simulink library "line_tracking_algorithm_atomic_sub_chart_library"  (R2013b)
settings: Solver=ode45  StartTime=0.0  StopTime=10.0  RelTol=1e-3
undefined symbols (not defined in the file): DiscIntNeverNeededParam, gcbh, realtime
libraries: legonxtlib x15, simulink x15
(part 1 of 2)
settings Model: Creator=mbiesiad  LastModifiedBy=menkh

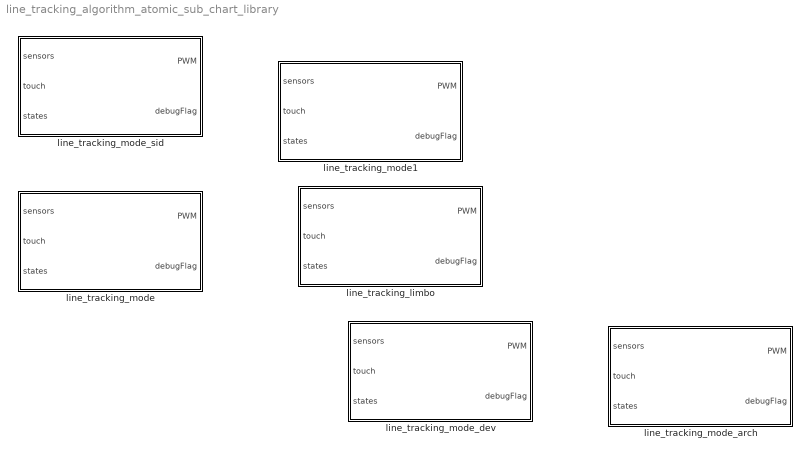
== system line_tracking_algorithm_atomic_sub_chart_library ==
  line_tracking_limbo : Stateflow chart  TreatAsAtomicUnit=on
  line_tracking_mode : Stateflow chart  TreatAsAtomicUnit=on
  line_tracking_mode1 : Stateflow chart  TreatAsAtomicUnit=on
  line_tracking_mode_arch : Stateflow chart  TreatAsAtomicUnit=on
  line_tracking_mode_dev : Stateflow chart  TreatAsAtomicUnit=on
  line_tracking_mode_sid : Stateflow chart  TreatAsAtomicUnit=on

== system line_tracking_algorithm_atomic_sub_chart_library/line_tracking_limbo/line_tracking_mode.DispTheta ==
  theta : Inport  OutDataTypeStr=double  PortDimensions=1
  f : TriggerPort  TriggerType=function-call
      settings: CopyFcn=Stateflow.SLINSF.SimulinkMan.removeBlockPreDeleteFcn  PreDeleteFcn=Stateflow.SLINSF.SimulinkMan.unsafePredeleteFcn
  Gain : Gain  Gain=10
  LCD : legonxtlib/LCD  slcdStr=Theta  slcdLine=2  slcdFormat=Decimal
  wires:
  theta/1 -> Gain/1
  Gain/1 -> LCD/1

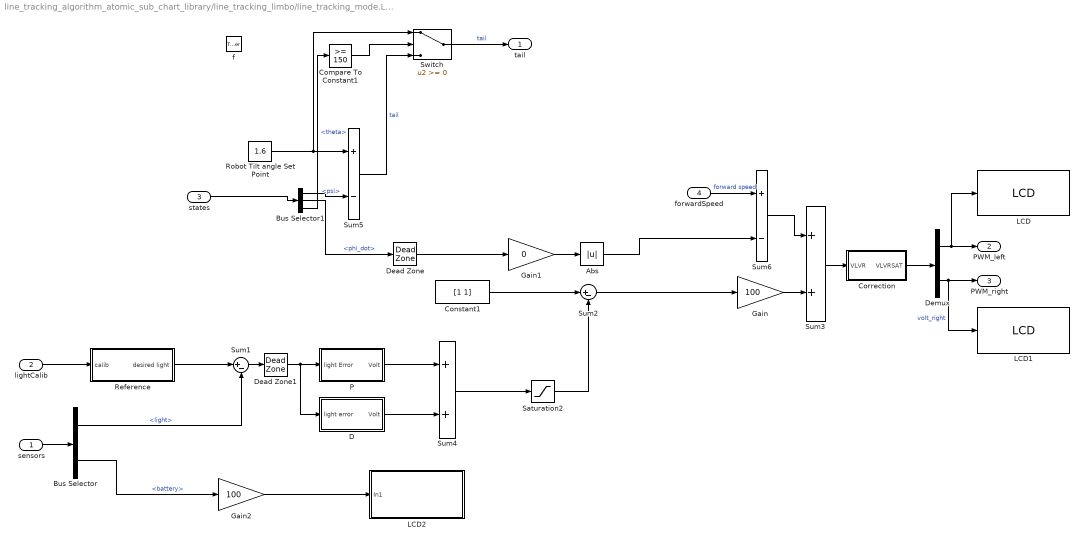
== system line_tracking_algorithm_atomic_sub_chart_library/line_tracking_limbo/line_tracking_mode.LineTrackAltFcn ==
  sensors : Inport  OutDataTypeStr=Bus: Sensors_Bus  PortDimensions=1
  lightCalib : Inport  Port=2  OutDataTypeStr=Bus: Light_Bus  PortDimensions=1
  states : Inport  Port=3  OutDataTypeStr=Bus: States_Bus  PortDimensions=1
  forwardSpeed : Inport  Port=4  OutDataTypeStr=single  PortDimensions=1
  f : TriggerPort  TriggerType=function-call
      settings: CopyFcn=Stateflow.SLINSF.SimulinkMan.removeBlockPreDeleteFcn  PreDeleteFcn=Stateflow.SLINSF.SimulinkMan.unsafePredeleteFcn
  Abs : Abs
  Bus Selector : BusSelector  OutputSignals=light,battery
  Bus Selector1 : BusSelector  OutputSignals=balancerStates.psi,phi_dot,balancerStates.theta
  Compare To Constant1 : simulink/Logic and Bit Operations/Compare To Constant  relop=>=  const=150  OutDataTypeStr=boolean
  Constant1 : Constant  Value=[1 1]  OutDataTypeStr=single
  Correction : Subsystem
  D : Subsystem
  Dead Zone : DeadZone  LowerValue=-3  UpperValue=3  SaturateOnIntegerOverflow=on
  Dead Zone1 : DeadZone  LowerValue=-0.1  UpperValue=0  SaturateOnIntegerOverflow=on
  Demux : Demux  Outputs=2
  Gain : Gain  Gain=100
  Gain1 : Gain  Gain=0
  Gain2 : Gain  Gain=100
  LCD : legonxtlib/LCD  slcdStr=VL  slcdLine=3  slcdFormat=Decimal
  LCD1 : legonxtlib/LCD  slcdStr=VR  slcdLine=4  slcdFormat=Decimal
  LCD2 : Subsystem  InitFcn=realtime.validateBlock('LEGO MINDSTORMS NXT', gcbh, '')  mask(LEGO MINDSTORMS NXT LCD){slcdStr=Battery, slcdLine=8, slcdFormat=Decimal}
      mask prompts: slcdStr "Display label (maximum  8 characters):"; slcdLine "Display at line:"; slcdFormat "Display format:"
      mask help: Displays the numeric value from the block input port. The display truncates the input value to show only the integer portion. Use Display at line parameter to select the row. Use Display format parameter to select the format of the number: decimal or hexadecimal.
      mask init:
      | realtime.internal.nxtLcdSysCallback;
      mask Help: eval('realtime.helpView(''LEGO MINDSTORMS NXT'', ''legonxtlibnxtlcd'')')
      mask TypeOptions slcdLine: 1 | 2 | 3 | 4 | 5 | 6 | 7 | 8
      mask TypeOptions slcdFormat: Decimal | Hex
      mask Display:
      | [data, map]=imread('LCD.gif');pic=ind2rgb(data,map);image(pic,[0.32 0.25 0.35 0.55]);
      | lineText = sprintf('Line %d', slcdLine);
      | text(0.5, 0.15, lineText, 'horizontalAlignment', 'center');
      | port_label('input', 1, '');
      | color('blue');
      | text(0.65, 0.87, 'LEGO', 'horizontalAlignment', 'left');
  P : Subsystem
  Reference : Subsystem
  Robot Tilt angle Set Point : Constant  Value=1.6  OutDataTypeStr=single
  Saturation2 : Saturate  UpperLimit=1  LowerLimit=0.45
  Sum1 : Sum  Inputs=|+-
  Sum2 : Sum  Inputs=|+-
  Sum3 : Sum
  Sum4 : Sum
  Sum5 : Sum  Inputs=+-
  Sum6 : Sum  Inputs=+-
  Switch : Switch
  tail : Outport  OutDataTypeStr=single  InitialOutput=0
  PWM_left : Outport  Port=2  OutDataTypeStr=single  InitialOutput=0
  PWM_right : Outport  Port=3  OutDataTypeStr=single  InitialOutput=0
  wires:
  Gain2/1 -> LCD2/1(In1)
  Bus Selector1/3 -> Compare To Constant1/1  "<theta>"
  Compare To Constant1/1 -> Switch/2
  Correction/1(VLVRSAT) -> Demux/1
  Sum3/1 -> Correction/1(VLVR)
  Abs/1 -> Sum6/2
  Bus Selector1/2 -> Dead Zone/1  "<phi_dot>"
  Gain1/1 -> Abs/1
  Sum6/1 -> Sum3/1
  Gain/1 -> Sum3/2
  Sum2/1 -> Gain/1
  forwardSpeed/1 -> Sum6/1  "forward speed"
  D/1(Volt) -> Sum4/2
  P/1(Volt) -> Sum4/1
  Reference/1(desired light) -> Sum1/1
  lightCalib/1 -> Reference/1(calib)
  Constant1/1 -> Sum2/1
  Robot Tilt angle Set Point/1 -> Switch/1, Sum5/1
  Bus Selector1/1 -> Sum5/2  "<psi>"
  states/1 -> Bus Selector1/1
  Sum4/1 -> Saturation2/1
  Sum1/1 -> Dead Zone1/1
  Saturation2/1 -> Sum2/2
  Bus Selector/1 -> Sum1/2  "<light>"
  sensors/1 -> Bus Selector/1
  Switch/1 -> tail/1  "tail"
  Demux/1 -> LCD/1, PWM_left/1
  Demux/2 -> LCD1/1, PWM_right/1  "volt_right"
  Dead Zone/1 -> Gain1/1
  Dead Zone1/1 -> P/1(light Error), D/1(light error)
  Sum5/1 -> Switch/3  "tail"
  Bus Selector/2 -> Gain2/1  "<battery>"

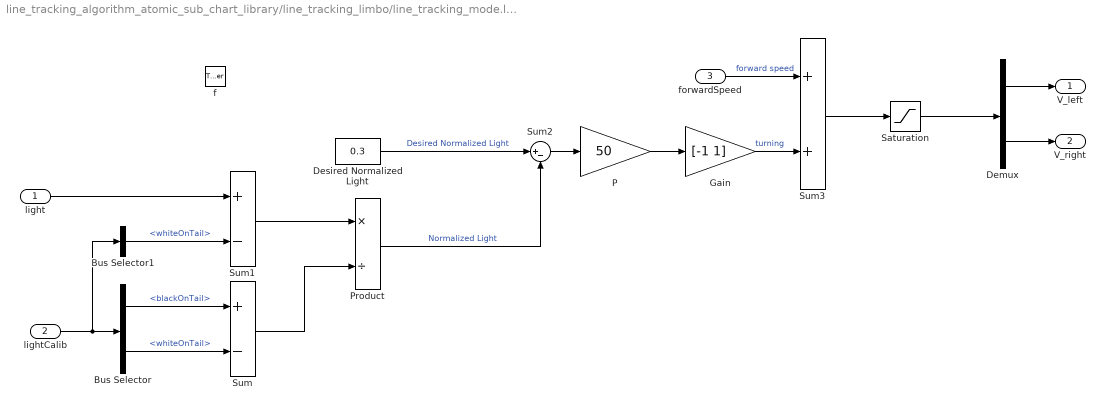
== system line_tracking_algorithm_atomic_sub_chart_library/line_tracking_limbo/line_tracking_mode.lineTrack ==
  light : Inport  OutDataTypeStr=single  PortDimensions=1
  lightCalib : Inport  Port=2  OutDataTypeStr=Bus: Light_Bus  PortDimensions=1
  forwardSpeed : Inport  Port=3  OutDataTypeStr=single  PortDimensions=1
  f : TriggerPort  TriggerType=function-call
      settings: CopyFcn=Stateflow.SLINSF.SimulinkMan.removeBlockPreDeleteFcn  PreDeleteFcn=Stateflow.SLINSF.SimulinkMan.unsafePredeleteFcn
  Bus Selector : BusSelector  OutputSignals=blackOnTail,whiteOnTail
  Bus Selector1 : BusSelector  OutputSignals=whiteOnTail
  Demux : Demux  Outputs=2
  Desired Normalized Light : Constant  Value=0.3  OutDataTypeStr=single
  Gain : Gain  Gain=[-1 1]
  P : Gain  Gain=50
  Product : Product  Inputs=*/
  Saturation : Saturate  UpperLimit=100  LowerLimit=-100  OutDataTypeStr=single
  Sum : Sum  Inputs=+-
  Sum1 : Sum  Inputs=+-
  Sum2 : Sum  Inputs=|+-
  Sum3 : Sum
  V_left : Outport  OutDataTypeStr=single  PortDimensions=1
  V_right : Outport  Port=2  OutDataTypeStr=single  PortDimensions=1
  wires:
  Saturation/1 -> Demux/1
  P/1 -> Gain/1
  Sum3/1 -> Saturation/1
  forwardSpeed/1 -> Sum3/1  "forward speed"
  Demux/2 -> V_right/1
  Demux/1 -> V_left/1
  Gain/1 -> Sum3/2  "turning"
  Sum2/1 -> P/1
  Desired Normalized Light/1 -> Sum2/1  "Desired Normalized Light"
  Product/1 -> Sum2/2  "Normalized Light"
  Sum1/1 -> Product/1
  Bus Selector1/1 -> Sum1/2  "<whiteOnTail>"
  light/1 -> Sum1/1
  Sum/1 -> Product/2
  Bus Selector/1 -> Sum/1  "<blackOnTail>"
  Bus Selector/2 -> Sum/2  "<whiteOnTail>"
  lightCalib/1 -> Bus Selector/1, Bus Selector1/1

== system line_tracking_algorithm_atomic_sub_chart_library/line_tracking_limbo/line_tracking_mode.tail_controller ==
  note: Could be improved, PI for example
  current : Inport  OutDataTypeStr=single  PortDimensions=1
  desired : Inport  Port=2  OutDataTypeStr=single  PortDimensions=1
  f : TriggerPort  TriggerType=function-call
      settings: CopyFcn=Stateflow.SLINSF.SimulinkMan.removeBlockPreDeleteFcn  PreDeleteFcn=Stateflow.SLINSF.SimulinkMan.unsafePredeleteFcn
  Gain : Gain  Gain=250
  Saturation : Saturate  UpperLimit=100  LowerLimit=-100  OutDataTypeStr=single
  Sum : Sum  Inputs=|+-
  cmd : Outport  OutDataTypeStr=single  PortDimensions=1  InitialOutput=0
  wires:
  Saturation/1 -> cmd/1
  Gain/1 -> Saturation/1
  desired/1 -> Sum/1
  current/1 -> Sum/2
  Sum/1 -> Gain/1

== system line_tracking_algorithm_atomic_sub_chart_library/line_tracking_mode/line_tracking_mode.DispTheta ==
  theta : Inport  OutDataTypeStr=double  PortDimensions=1
  f : TriggerPort  TriggerType=function-call
      settings: CopyFcn=Stateflow.SLINSF.SimulinkMan.removeBlockPreDeleteFcn  PreDeleteFcn=Stateflow.SLINSF.SimulinkMan.unsafePredeleteFcn
  Gain : Gain  Gain=10
  LCD : legonxtlib/LCD  slcdStr=Theta  slcdLine=2  slcdFormat=Decimal
  wires:
  theta/1 -> Gain/1
  Gain/1 -> LCD/1

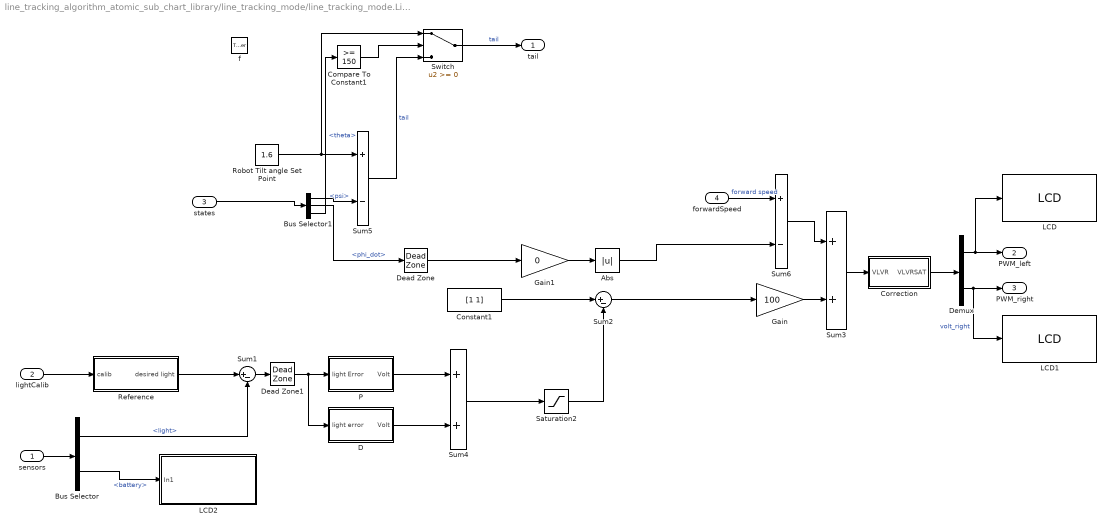
== system line_tracking_algorithm_atomic_sub_chart_library/line_tracking_mode/line_tracking_mode.LineTrackAltFcn ==
  sensors : Inport  OutDataTypeStr=Bus: Sensors_Bus  PortDimensions=1
  lightCalib : Inport  Port=2  OutDataTypeStr=Bus: Light_Bus  PortDimensions=1
  states : Inport  Port=3  OutDataTypeStr=Bus: States_Bus  PortDimensions=1
  forwardSpeed : Inport  Port=4  OutDataTypeStr=single  PortDimensions=1
  f : TriggerPort  TriggerType=function-call
      settings: CopyFcn=Stateflow.SLINSF.SimulinkMan.removeBlockPreDeleteFcn  PreDeleteFcn=Stateflow.SLINSF.SimulinkMan.unsafePredeleteFcn
  Abs : Abs
  Bus Selector : BusSelector  OutputSignals=light,battery
  Bus Selector1 : BusSelector  OutputSignals=balancerStates.psi,phi_dot,balancerStates.theta
  Compare To Constant1 : simulink/Logic and Bit Operations/Compare To Constant  relop=>=  const=150  OutDataTypeStr=boolean
  Constant1 : Constant  Value=[1 1]  OutDataTypeStr=single
  Correction : Subsystem
  D : Subsystem
  Dead Zone : DeadZone  LowerValue=-3  UpperValue=3  SaturateOnIntegerOverflow=on
  Dead Zone1 : DeadZone  LowerValue=-0.1  UpperValue=0  SaturateOnIntegerOverflow=on
  Demux : Demux  Outputs=2
  Gain : Gain  Gain=100
  Gain1 : Gain  Gain=0
  LCD : legonxtlib/LCD  slcdStr=VL  slcdLine=3  slcdFormat=Decimal
  LCD1 : legonxtlib/LCD  slcdStr=VR  slcdLine=4  slcdFormat=Decimal
  LCD2 : Subsystem  InitFcn=realtime.validateBlock('LEGO MINDSTORMS NXT', gcbh, '')  mask(LEGO MINDSTORMS NXT LCD){slcdStr=Battery, slcdLine=8, slcdFormat=Decimal}
      mask prompts: slcdStr "Display label (maximum  8 characters):"; slcdLine "Display at line:"; slcdFormat "Display format:"
      mask help: Displays the numeric value from the block input port. The display truncates the input value to show only the integer portion. Use Display at line parameter to select the row. Use Display format parameter to select the format of the number: decimal or hexadecimal.
      mask init:
      | realtime.internal.nxtLcdSysCallback;
      mask Help: eval('realtime.helpView(''LEGO MINDSTORMS NXT'', ''legonxtlibnxtlcd'')')
      mask TypeOptions slcdLine: 1 | 2 | 3 | 4 | 5 | 6 | 7 | 8
      mask TypeOptions slcdFormat: Decimal | Hex
      mask Display:
      | [data, map]=imread('LCD.gif');pic=ind2rgb(data,map);image(pic,[0.32 0.25 0.35 0.55]);
      | lineText = sprintf('Line %d', slcdLine);
      | text(0.5, 0.15, lineText, 'horizontalAlignment', 'center');
      | port_label('input', 1, '');
      | color('blue');
      | text(0.65, 0.87, 'LEGO', 'horizontalAlignment', 'left');
  P : Subsystem
  Reference : Subsystem
  Robot Tilt angle Set Point : Constant  Value=1.6  OutDataTypeStr=single
  Saturation2 : Saturate  UpperLimit=1  LowerLimit=0.45
  Sum1 : Sum  Inputs=|+-
  Sum2 : Sum  Inputs=|+-
  Sum3 : Sum
  Sum4 : Sum
  Sum5 : Sum  Inputs=+-
  Sum6 : Sum  Inputs=+-
  Switch : Switch
  tail : Outport  OutDataTypeStr=single  InitialOutput=0
  PWM_left : Outport  Port=2  OutDataTypeStr=single  InitialOutput=0
  PWM_right : Outport  Port=3  OutDataTypeStr=single  InitialOutput=0
  wires:
  Bus Selector1/3 -> Compare To Constant1/1  "<theta>"
  Compare To Constant1/1 -> Switch/2
  Correction/1(VLVRSAT) -> Demux/1
  Sum3/1 -> Correction/1(VLVR)
  Abs/1 -> Sum6/2
  Bus Selector1/2 -> Dead Zone/1  "<phi_dot>"
  Gain1/1 -> Abs/1
  Sum6/1 -> Sum3/1
  Gain/1 -> Sum3/2
  Sum2/1 -> Gain/1
  forwardSpeed/1 -> Sum6/1  "forward speed"
  D/1(Volt) -> Sum4/2
  P/1(Volt) -> Sum4/1
  Reference/1(desired light) -> Sum1/1
  lightCalib/1 -> Reference/1(calib)
  Constant1/1 -> Sum2/1
  Robot Tilt angle Set Point/1 -> Switch/1, Sum5/1
  Bus Selector1/1 -> Sum5/2  "<psi>"
  states/1 -> Bus Selector1/1
  Sum4/1 -> Saturation2/1
  Sum1/1 -> Dead Zone1/1
  Saturation2/1 -> Sum2/2
  Bus Selector/1 -> Sum1/2  "<light>"
  sensors/1 -> Bus Selector/1
  Switch/1 -> tail/1  "tail"
  Demux/1 -> LCD/1, PWM_left/1
  Demux/2 -> LCD1/1, PWM_right/1  "volt_right"
  Dead Zone/1 -> Gain1/1
  Dead Zone1/1 -> P/1(light Error), D/1(light error)
  Sum5/1 -> Switch/3  "tail"
  Bus Selector/2 -> LCD2/1(In1)  "<battery>"

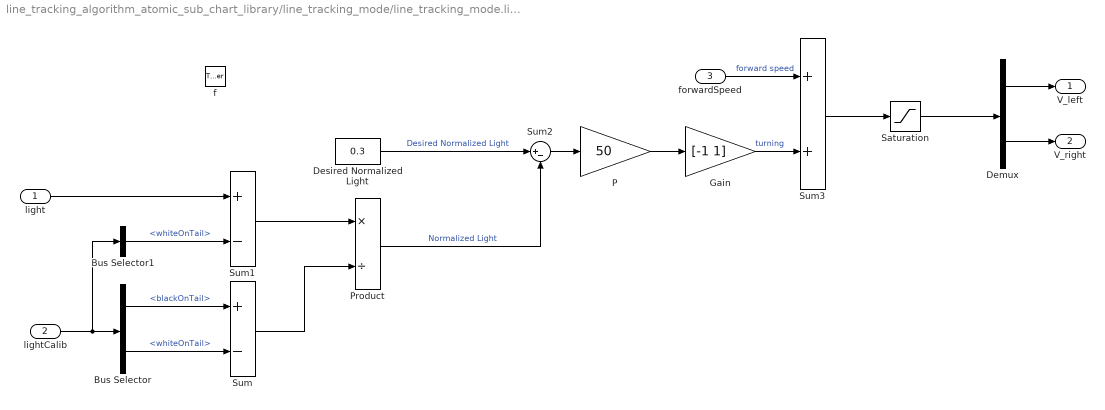
== system line_tracking_algorithm_atomic_sub_chart_library/line_tracking_mode/line_tracking_mode.lineTrack ==
  light : Inport  OutDataTypeStr=single  PortDimensions=1
  lightCalib : Inport  Port=2  OutDataTypeStr=Bus: Light_Bus  PortDimensions=1
  forwardSpeed : Inport  Port=3  OutDataTypeStr=single  PortDimensions=1
  f : TriggerPort  TriggerType=function-call
      settings: CopyFcn=Stateflow.SLINSF.SimulinkMan.removeBlockPreDeleteFcn  PreDeleteFcn=Stateflow.SLINSF.SimulinkMan.unsafePredeleteFcn
  Bus Selector : BusSelector  OutputSignals=blackOnTail,whiteOnTail
  Bus Selector1 : BusSelector  OutputSignals=whiteOnTail
  Demux : Demux  Outputs=2
  Desired Normalized Light : Constant  Value=0.3  OutDataTypeStr=single
  Gain : Gain  Gain=[-1 1]
  P : Gain  Gain=50
  Product : Product  Inputs=*/
  Saturation : Saturate  UpperLimit=100  LowerLimit=-100  OutDataTypeStr=single
  Sum : Sum  Inputs=+-
  Sum1 : Sum  Inputs=+-
  Sum2 : Sum  Inputs=|+-
  Sum3 : Sum
  V_left : Outport  OutDataTypeStr=single  PortDimensions=1
  V_right : Outport  Port=2  OutDataTypeStr=single  PortDimensions=1
  wires:
  Saturation/1 -> Demux/1
  P/1 -> Gain/1
  Sum3/1 -> Saturation/1
  forwardSpeed/1 -> Sum3/1  "forward speed"
  Demux/2 -> V_right/1
  Demux/1 -> V_left/1
  Gain/1 -> Sum3/2  "turning"
  Sum2/1 -> P/1
  Desired Normalized Light/1 -> Sum2/1  "Desired Normalized Light"
  Product/1 -> Sum2/2  "Normalized Light"
  Sum1/1 -> Product/1
  Bus Selector1/1 -> Sum1/2  "<whiteOnTail>"
  light/1 -> Sum1/1
  Sum/1 -> Product/2
  Bus Selector/1 -> Sum/1  "<blackOnTail>"
  Bus Selector/2 -> Sum/2  "<whiteOnTail>"
  lightCalib/1 -> Bus Selector/1, Bus Selector1/1

== system line_tracking_algorithm_atomic_sub_chart_library/line_tracking_mode/line_tracking_mode.tail_controller ==
  note: Could be improved, PI for example
  current : Inport  OutDataTypeStr=single  PortDimensions=1
  desired : Inport  Port=2  OutDataTypeStr=single  PortDimensions=1
  f : TriggerPort  TriggerType=function-call
      settings: CopyFcn=Stateflow.SLINSF.SimulinkMan.removeBlockPreDeleteFcn  PreDeleteFcn=Stateflow.SLINSF.SimulinkMan.unsafePredeleteFcn
  Gain : Gain  Gain=250
  Saturation : Saturate  UpperLimit=100  LowerLimit=-100  OutDataTypeStr=single
  Sum : Sum  Inputs=|+-
  cmd : Outport  OutDataTypeStr=single  PortDimensions=1  InitialOutput=0
  wires:
  Saturation/1 -> cmd/1
  Gain/1 -> Saturation/1
  desired/1 -> Sum/1
  current/1 -> Sum/2
  Sum/1 -> Gain/1

== system line_tracking_algorithm_atomic_sub_chart_library/line_tracking_mode1/line_tracking_mode.DispTheta ==
  theta : Inport  OutDataTypeStr=double  PortDimensions=1
  f : TriggerPort  TriggerType=function-call
      settings: CopyFcn=Stateflow.SLINSF.SimulinkMan.removeBlockPreDeleteFcn  PreDeleteFcn=Stateflow.SLINSF.SimulinkMan.unsafePredeleteFcn
  Gain : Gain  Gain=10
  LCD : legonxtlib/LCD  slcdStr=Theta  slcdLine=2  slcdFormat=Decimal
  wires:
  Gain/1 -> LCD/1
  theta/1 -> Gain/1

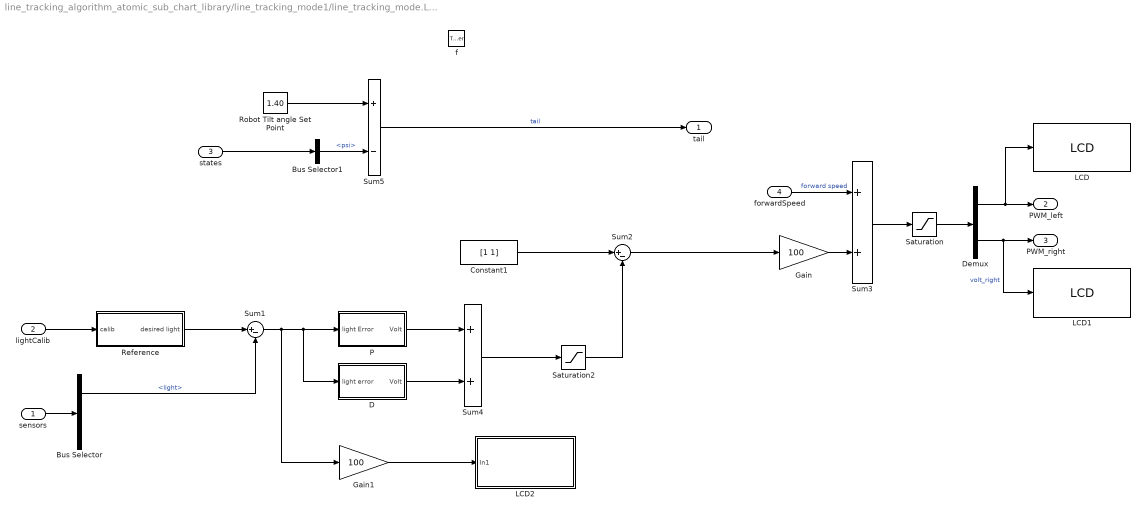
== system line_tracking_algorithm_atomic_sub_chart_library/line_tracking_mode1/line_tracking_mode.LineTrackAltFcn ==
  sensors : Inport  OutDataTypeStr=Bus: Sensors_Bus  PortDimensions=1
  lightCalib : Inport  Port=2  OutDataTypeStr=Bus: Light_Bus  PortDimensions=1
  states : Inport  Port=3  OutDataTypeStr=Bus: Balancer_States_Bus  PortDimensions=1
  forwardSpeed : Inport  Port=4  OutDataTypeStr=single  PortDimensions=1
  f : TriggerPort  TriggerType=function-call
      settings: CopyFcn=Stateflow.SLINSF.SimulinkMan.removeBlockPreDeleteFcn  PreDeleteFcn=Stateflow.SLINSF.SimulinkMan.unsafePredeleteFcn
  Bus Selector : BusSelector  OutputSignals=light,battery
  Bus Selector1 : BusSelector  OutputSignals=psi
  Constant1 : Constant  Value=[1 1]  OutDataTypeStr=single
  D : Subsystem
  Demux : Demux  Outputs=2
  Gain : Gain  Gain=100
  Gain1 : Gain  Gain=100
  LCD : legonxtlib/LCD  slcdStr=VL  slcdLine=3  slcdFormat=Decimal
  LCD1 : legonxtlib/LCD  slcdStr=VR  slcdLine=4  slcdFormat=Decimal
  LCD2 : Subsystem  InitFcn=realtime.validateBlock('LEGO MINDSTORMS NXT', gcbh, '')  mask(LEGO MINDSTORMS NXT LCD){slcdStr=Lerror, slcdLine=5, slcdFormat=Decimal}
      mask prompts: slcdStr "Display label (maximum  8 characters):"; slcdLine "Display at line:"; slcdFormat "Display format:"
      mask help: Displays the numeric value from the block input port. The display truncates the input value to show only the integer portion. Use Display at line parameter to select the row. Use Display format parameter to select the format of the number: decimal or hexadecimal.
      mask init:
      | realtime.internal.nxtLcdSysCallback;
      mask Help: eval('realtime.helpView(''LEGO MINDSTORMS NXT'', ''legonxtlibnxtlcd'')')
      mask TypeOptions slcdLine: 1 | 2 | 3 | 4 | 5 | 6 | 7 | 8
      mask TypeOptions slcdFormat: Decimal | Hex
      mask Display:
      | [data, map]=imread('LCD.gif');pic=ind2rgb(data,map);image(pic,[0.32 0.25 0.35 0.55]);
      | lineText = sprintf('Line %d', slcdLine);
      | text(0.5, 0.15, lineText, 'horizontalAlignment', 'center');
      | port_label('input', 1, '');
      | color('blue');
      | text(0.65, 0.87, 'LEGO', 'horizontalAlignment', 'left');
  P : Subsystem
  Reference : Subsystem
  Robot Tilt angle Set Point : Constant  Value=1.40  OutDataTypeStr=single
  Saturation : Saturate  UpperLimit=100  LowerLimit=-100  OutDataTypeStr=single
  Saturation2 : Saturate  UpperLimit=1  LowerLimit=0.6
  Sum1 : Sum  Inputs=|+-
  Sum2 : Sum  Inputs=|+-
  Sum3 : Sum
  Sum4 : Sum
  Sum5 : Sum  Inputs=+-
  tail : Outport  OutDataTypeStr=single  InitialOutput=0
  PWM_left : Outport  Port=2  OutDataTypeStr=single  InitialOutput=0
  PWM_right : Outport  Port=3  OutDataTypeStr=single  InitialOutput=0
  wires:
  Gain1/1 -> LCD2/1(In1)
  Demux/2 -> PWM_right/1, LCD1/1  "volt_right"
  Demux/1 -> PWM_left/1, LCD/1
  Sum5/1 -> tail/1  "tail"
  sensors/1 -> Bus Selector/1
  Bus Selector/1 -> Sum1/2  "<light>"
  Saturation2/1 -> Sum2/2
  Sum1/1 -> D/1(light error), P/1(light Error), Gain1/1
  Sum4/1 -> Saturation2/1
  states/1 -> Bus Selector1/1
  Bus Selector1/1 -> Sum5/2  "<psi>"
  Robot Tilt angle Set Point/1 -> Sum5/1
  Constant1/1 -> Sum2/1
  lightCalib/1 -> Reference/1(calib)
  Reference/1(desired light) -> Sum1/1
  P/1(Volt) -> Sum4/1
  D/1(Volt) -> Sum4/2
  forwardSpeed/1 -> Sum3/1  "forward speed"
  Sum3/1 -> Saturation/1
  Saturation/1 -> Demux/1
  Sum2/1 -> Gain/1
  Gain/1 -> Sum3/2

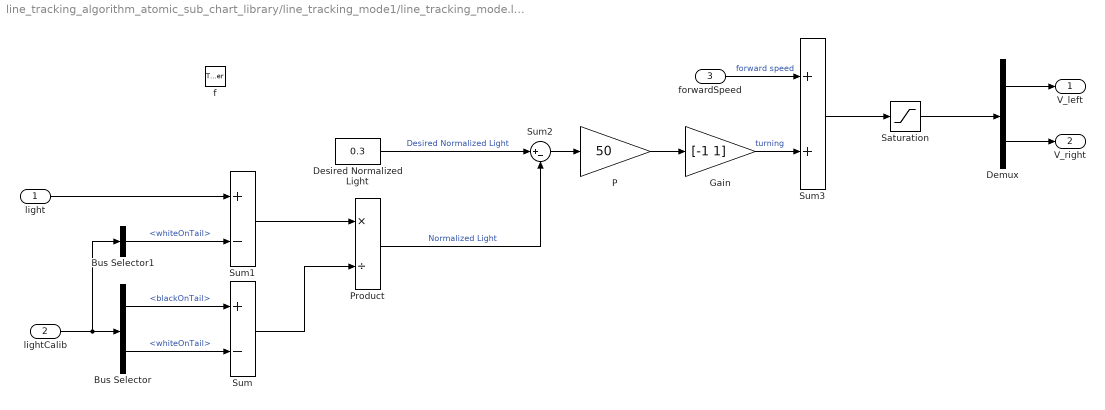
== system line_tracking_algorithm_atomic_sub_chart_library/line_tracking_mode1/line_tracking_mode.lineTrack ==
  light : Inport  OutDataTypeStr=single  PortDimensions=1
  lightCalib : Inport  Port=2  OutDataTypeStr=Bus: Light_Bus  PortDimensions=1
  forwardSpeed : Inport  Port=3  OutDataTypeStr=single  PortDimensions=1
  f : TriggerPort  TriggerType=function-call
      settings: CopyFcn=Stateflow.SLINSF.SimulinkMan.removeBlockPreDeleteFcn  PreDeleteFcn=Stateflow.SLINSF.SimulinkMan.unsafePredeleteFcn
  Bus Selector : BusSelector  OutputSignals=blackOnTail,whiteOnTail
  Bus Selector1 : BusSelector  OutputSignals=whiteOnTail
  Demux : Demux  Outputs=2
  Desired Normalized Light : Constant  Value=0.3  OutDataTypeStr=single
  Gain : Gain  Gain=[-1 1]
  P : Gain  Gain=50
  Product : Product  Inputs=*/
  Saturation : Saturate  UpperLimit=100  LowerLimit=-100  OutDataTypeStr=single
  Sum : Sum  Inputs=+-
  Sum1 : Sum  Inputs=+-
  Sum2 : Sum  Inputs=|+-
  Sum3 : Sum
  V_left : Outport  OutDataTypeStr=single  PortDimensions=1
  V_right : Outport  Port=2  OutDataTypeStr=single  PortDimensions=1
  wires:
  lightCalib/1 -> Bus Selector1/1, Bus Selector/1
  Bus Selector/2 -> Sum/2  "<whiteOnTail>"
  Bus Selector/1 -> Sum/1  "<blackOnTail>"
  Sum/1 -> Product/2
  light/1 -> Sum1/1
  Bus Selector1/1 -> Sum1/2  "<whiteOnTail>"
  Sum1/1 -> Product/1
  Product/1 -> Sum2/2  "Normalized Light"
  Desired Normalized Light/1 -> Sum2/1  "Desired Normalized Light"
  Sum2/1 -> P/1
  Gain/1 -> Sum3/2  "turning"
  Demux/1 -> V_left/1
  Demux/2 -> V_right/1
  forwardSpeed/1 -> Sum3/1  "forward speed"
  Sum3/1 -> Saturation/1
  P/1 -> Gain/1
  Saturation/1 -> Demux/1

== system line_tracking_algorithm_atomic_sub_chart_library/line_tracking_mode1/line_tracking_mode.tail_controller ==
  note: Could be improved, PI for example
  current : Inport  OutDataTypeStr=single  PortDimensions=1
  desired : Inport  Port=2  OutDataTypeStr=single  PortDimensions=1
  f : TriggerPort  TriggerType=function-call
      settings: CopyFcn=Stateflow.SLINSF.SimulinkMan.removeBlockPreDeleteFcn  PreDeleteFcn=Stateflow.SLINSF.SimulinkMan.unsafePredeleteFcn
  Gain : Gain  Gain=250
  Saturation : Saturate  UpperLimit=100  LowerLimit=-100  OutDataTypeStr=single
  Sum : Sum  Inputs=|+-
  cmd : Outport  OutDataTypeStr=single  PortDimensions=1  InitialOutput=0
  wires:
  Sum/1 -> Gain/1
  current/1 -> Sum/2
  desired/1 -> Sum/1
  Gain/1 -> Saturation/1
  Saturation/1 -> cmd/1

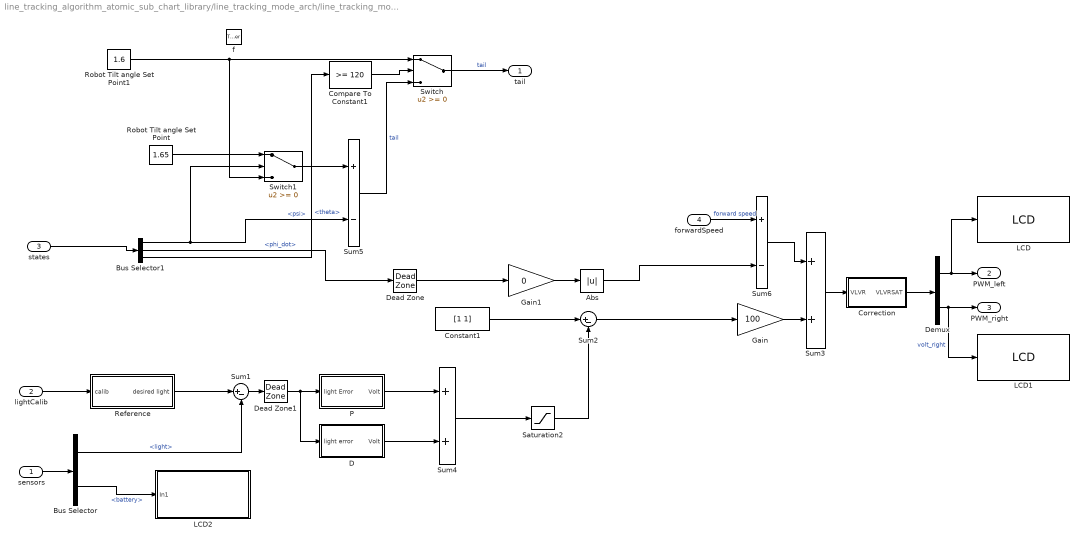
== system line_tracking_algorithm_atomic_sub_chart_library/line_tracking_mode_arch/line_tracking_mode.LineTrackAltFcn ==
  sensors : Inport  OutDataTypeStr=Bus: Sensors_Bus  PortDimensions=1
  lightCalib : Inport  Port=2  OutDataTypeStr=Bus: Light_Bus  PortDimensions=1
  states : Inport  Port=3  OutDataTypeStr=Bus: States_Bus  PortDimensions=1
  forwardSpeed : Inport  Port=4  OutDataTypeStr=single  PortDimensions=1
  f : TriggerPort  TriggerType=function-call
      settings: CopyFcn=Stateflow.SLINSF.SimulinkMan.removeBlockPreDeleteFcn  PreDeleteFcn=Stateflow.SLINSF.SimulinkMan.unsafePredeleteFcn
  Abs : Abs
  Bus Selector : BusSelector  OutputSignals=light,battery
  Bus Selector1 : BusSelector  OutputSignals=balancerStates.psi,phi_dot,balancerStates.theta
  Compare To Constant1 : simulink/Logic and Bit Operations/Compare To Constant  relop=>=  const=120  OutDataTypeStr=boolean
  Constant1 : Constant  Value=[1 1]  OutDataTypeStr=single
  Correction : Subsystem
  D : Subsystem
  Dead Zone : DeadZone  LowerValue=-3  UpperValue=3  SaturateOnIntegerOverflow=on
  Dead Zone1 : DeadZone  LowerValue=-0.1  UpperValue=0  SaturateOnIntegerOverflow=on
  Demux : Demux  Outputs=2
  Gain : Gain  Gain=100
  Gain1 : Gain  Gain=0
  LCD : legonxtlib/LCD  slcdStr=VL  slcdLine=3  slcdFormat=Decimal
  LCD1 : legonxtlib/LCD  slcdStr=VR  slcdLine=4  slcdFormat=Decimal
  LCD2 : Subsystem  InitFcn=realtime.validateBlock('LEGO MINDSTORMS NXT', gcbh, '')  mask(LEGO MINDSTORMS NXT LCD){slcdStr=Battery, slcdLine=8, slcdFormat=Decimal}
      mask prompts: slcdStr "Display label (maximum  8 characters):"; slcdLine "Display at line:"; slcdFormat "Display format:"
      mask help: Displays the numeric value from the block input port. The display truncates the input value to show only the integer portion. Use Display at line parameter to select the row. Use Display format parameter to select the format of the number: decimal or hexadecimal.
      mask init:
      | realtime.internal.nxtLcdSysCallback;
      mask Help: eval('realtime.helpView(''LEGO MINDSTORMS NXT'', ''legonxtlibnxtlcd'')')
      mask TypeOptions slcdLine: 1 | 2 | 3 | 4 | 5 | 6 | 7 | 8
      mask TypeOptions slcdFormat: Decimal | Hex
      mask Display:
      | [data, map]=imread('LCD.gif');pic=ind2rgb(data,map);image(pic,[0.32 0.25 0.35 0.55]);
      | lineText = sprintf('Line %d', slcdLine);
      | text(0.5, 0.15, lineText, 'horizontalAlignment', 'center');
      | port_label('input', 1, '');
      | color('blue');
      | text(0.65, 0.87, 'LEGO', 'horizontalAlignment', 'left');
  P : Subsystem
  Reference : Subsystem
  Robot Tilt angle Set Point : Constant  Value=1.65  OutDataTypeStr=single
  Robot Tilt angle Set Point1 : Constant  Value=1.6  OutDataTypeStr=single
  Saturation2 : Saturate  UpperLimit=1  LowerLimit=0.45
  Sum1 : Sum  Inputs=|+-
  Sum2 : Sum  Inputs=|+-
  Sum3 : Sum
  Sum4 : Sum
  Sum5 : Sum  Inputs=+-
  Sum6 : Sum  Inputs=+-
  Switch : Switch
  Switch1 : Switch
  tail : Outport  OutDataTypeStr=single  InitialOutput=0
  PWM_left : Outport  Port=2  OutDataTypeStr=single  InitialOutput=0
  PWM_right : Outport  Port=3  OutDataTypeStr=single  InitialOutput=0
  wires:
  Bus Selector/2 -> LCD2/1(In1)  "<battery>"
  Sum5/1 -> Switch/3  "tail"
  Dead Zone1/1 -> D/1(light error), P/1(light Error)
  Dead Zone/1 -> Gain1/1
  Demux/2 -> PWM_right/1, LCD1/1  "volt_right"
  Demux/1 -> PWM_left/1, LCD/1
  Switch/1 -> tail/1  "tail"
  sensors/1 -> Bus Selector/1
  Bus Selector/1 -> Sum1/2  "<light>"
  Saturation2/1 -> Sum2/2
  Sum1/1 -> Dead Zone1/1
  Sum4/1 -> Saturation2/1
  states/1 -> Bus Selector1/1
  Bus Selector1/1 -> Switch1/2, Sum5/2  "<psi>"
  Robot Tilt angle Set Point/1 -> Switch1/1
  Constant1/1 -> Sum2/1
  lightCalib/1 -> Reference/1(calib)
  Reference/1(desired light) -> Sum1/1
  P/1(Volt) -> Sum4/1
  D/1(Volt) -> Sum4/2
  forwardSpeed/1 -> Sum6/1  "forward speed"
  Sum2/1 -> Gain/1
  Gain/1 -> Sum3/2
  Sum6/1 -> Sum3/1
  Gain1/1 -> Abs/1
  Bus Selector1/2 -> Dead Zone/1  "<phi_dot>"
  Abs/1 -> Sum6/2
  Sum3/1 -> Correction/1(VLVR)
  Correction/1(VLVRSAT) -> Demux/1
  Compare To Constant1/1 -> Switch/2
  Bus Selector1/3 -> Compare To Constant1/1  "<theta>"
  Robot Tilt angle Set Point1/1 -> Switch1/3, Switch/1
  Switch1/1 -> Sum5/1

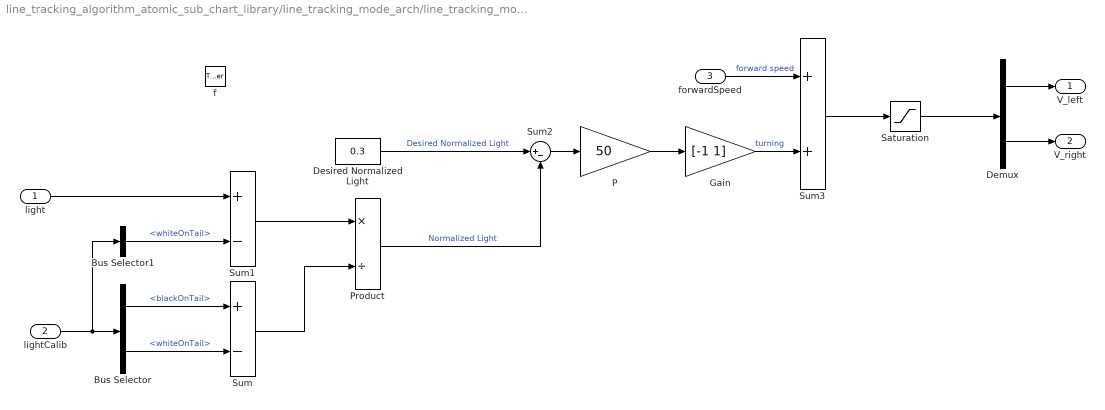
== system line_tracking_algorithm_atomic_sub_chart_library/line_tracking_mode_arch/line_tracking_mode.lineTrack ==
  light : Inport  OutDataTypeStr=single  PortDimensions=1
  lightCalib : Inport  Port=2  OutDataTypeStr=Bus: Light_Bus  PortDimensions=1
  forwardSpeed : Inport  Port=3  OutDataTypeStr=single  PortDimensions=1
  f : TriggerPort  TriggerType=function-call
      settings: CopyFcn=Stateflow.SLINSF.SimulinkMan.removeBlockPreDeleteFcn  PreDeleteFcn=Stateflow.SLINSF.SimulinkMan.unsafePredeleteFcn
  Bus Selector : BusSelector  OutputSignals=blackOnTail,whiteOnTail
  Bus Selector1 : BusSelector  OutputSignals=whiteOnTail
  Demux : Demux  Outputs=2
  Desired Normalized Light : Constant  Value=0.3  OutDataTypeStr=single
  Gain : Gain  Gain=[-1 1]
  P : Gain  Gain=50
  Product : Product  Inputs=*/
  Saturation : Saturate  UpperLimit=100  LowerLimit=-100  OutDataTypeStr=single
  Sum : Sum  Inputs=+-
  Sum1 : Sum  Inputs=+-
  Sum2 : Sum  Inputs=|+-
  Sum3 : Sum
  V_left : Outport  OutDataTypeStr=single  PortDimensions=1
  V_right : Outport  Port=2  OutDataTypeStr=single  PortDimensions=1
  wires:
  lightCalib/1 -> Bus Selector1/1, Bus Selector/1
  Bus Selector/2 -> Sum/2  "<whiteOnTail>"
  Bus Selector/1 -> Sum/1  "<blackOnTail>"
  Sum/1 -> Product/2
  light/1 -> Sum1/1
  Bus Selector1/1 -> Sum1/2  "<whiteOnTail>"
  Sum1/1 -> Product/1
  Product/1 -> Sum2/2  "Normalized Light"
  Desired Normalized Light/1 -> Sum2/1  "Desired Normalized Light"
  Sum2/1 -> P/1
  Gain/1 -> Sum3/2  "turning"
  Demux/1 -> V_left/1
  Demux/2 -> V_right/1
  forwardSpeed/1 -> Sum3/1  "forward speed"
  Sum3/1 -> Saturation/1
  P/1 -> Gain/1
  Saturation/1 -> Demux/1

== system line_tracking_algorithm_atomic_sub_chart_library/line_tracking_mode_arch/line_tracking_mode.tail_controller ==
  note: Could be improved, PI for example
  current : Inport  OutDataTypeStr=single  PortDimensions=1
  desired : Inport  Port=2  OutDataTypeStr=single  PortDimensions=1
  f : TriggerPort  TriggerType=function-call
      settings: CopyFcn=Stateflow.SLINSF.SimulinkMan.removeBlockPreDeleteFcn  PreDeleteFcn=Stateflow.SLINSF.SimulinkMan.unsafePredeleteFcn
  Gain : Gain  Gain=250
  Saturation : Saturate  UpperLimit=100  LowerLimit=-100  OutDataTypeStr=single
  Sum : Sum  Inputs=|+-
  cmd : Outport  OutDataTypeStr=single  PortDimensions=1  InitialOutput=0
  wires:
  Sum/1 -> Gain/1
  current/1 -> Sum/2
  desired/1 -> Sum/1
  Gain/1 -> Saturation/1
  Saturation/1 -> cmd/1

== system line_tracking_algorithm_atomic_sub_chart_library/line_tracking_mode_dev/line_tracking_mode.DispTheta ==
  theta : Inport  OutDataTypeStr=double  PortDimensions=1
  f : TriggerPort  TriggerType=function-call
      settings: CopyFcn=Stateflow.SLINSF.SimulinkMan.removeBlockPreDeleteFcn  PreDeleteFcn=Stateflow.SLINSF.SimulinkMan.unsafePredeleteFcn
  Gain : Gain  Gain=10
  LCD : legonxtlib/LCD  slcdStr=Theta  slcdLine=2  slcdFormat=Decimal
  wires:
  Gain/1 -> LCD/1
  theta/1 -> Gain/1

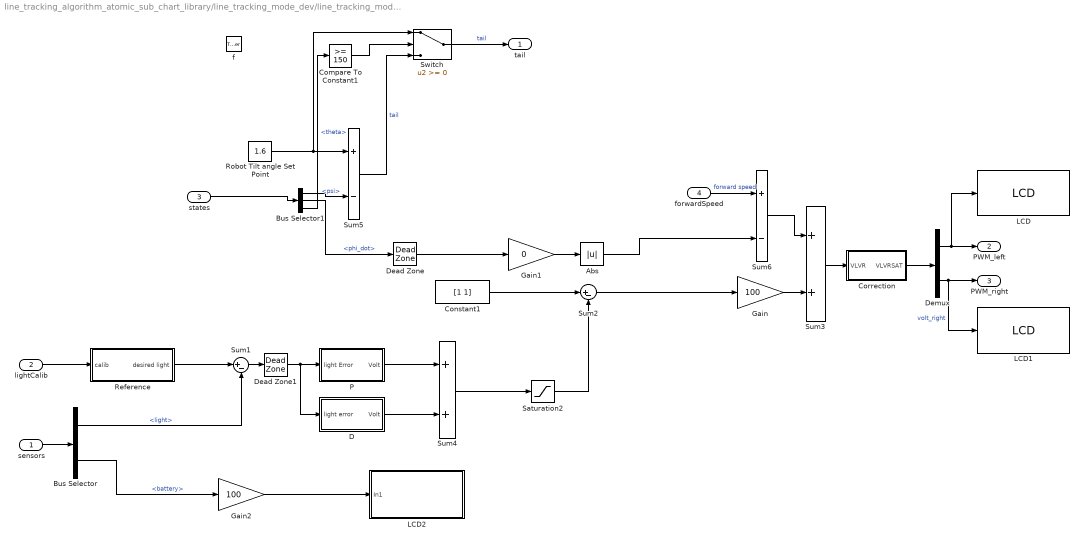
== system line_tracking_algorithm_atomic_sub_chart_library/line_tracking_mode_dev/line_tracking_mode.LineTrackAltFcn ==
  sensors : Inport  OutDataTypeStr=Bus: Sensors_Bus  PortDimensions=1
  lightCalib : Inport  Port=2  OutDataTypeStr=Bus: Light_Bus  PortDimensions=1
  states : Inport  Port=3  OutDataTypeStr=Bus: States_Bus  PortDimensions=1
  forwardSpeed : Inport  Port=4  OutDataTypeStr=single  PortDimensions=1
  f : TriggerPort  TriggerType=function-call
      settings: CopyFcn=Stateflow.SLINSF.SimulinkMan.removeBlockPreDeleteFcn  PreDeleteFcn=Stateflow.SLINSF.SimulinkMan.unsafePredeleteFcn
  Abs : Abs
  Bus Selector : BusSelector  OutputSignals=light,battery
  Bus Selector1 : BusSelector  OutputSignals=balancerStates.psi,phi_dot,balancerStates.theta
  Compare To Constant1 : simulink/Logic and Bit Operations/Compare To Constant  relop=>=  const=150  OutDataTypeStr=boolean
  Constant1 : Constant  Value=[1 1]  OutDataTypeStr=single
  Correction : Subsystem
  D : Subsystem
  Dead Zone : DeadZone  LowerValue=-3  UpperValue=3  SaturateOnIntegerOverflow=on
  Dead Zone1 : DeadZone  LowerValue=-0.1  UpperValue=0  SaturateOnIntegerOverflow=on
  Demux : Demux  Outputs=2
  Gain : Gain  Gain=100
  Gain1 : Gain  Gain=0
  Gain2 : Gain  Gain=100
  LCD : legonxtlib/LCD  slcdStr=VL  slcdLine=3  slcdFormat=Decimal
  LCD1 : legonxtlib/LCD  slcdStr=VR  slcdLine=4  slcdFormat=Decimal
  LCD2 : Subsystem  InitFcn=realtime.validateBlock('LEGO MINDSTORMS NXT', gcbh, '')  mask(LEGO MINDSTORMS NXT LCD){slcdStr=Battery, slcdLine=8, slcdFormat=Decimal}
      mask prompts: slcdStr "Display label (maximum  8 characters):"; slcdLine "Display at line:"; slcdFormat "Display format:"
      mask help: Displays the numeric value from the block input port. The display truncates the input value to show only the integer portion. Use Display at line parameter to select the row. Use Display format parameter to select the format of the number: decimal or hexadecimal.
      mask init:
      | realtime.internal.nxtLcdSysCallback;
      mask Help: eval('realtime.helpView(''LEGO MINDSTORMS NXT'', ''legonxtlibnxtlcd'')')
      mask TypeOptions slcdLine: 1 | 2 | 3 | 4 | 5 | 6 | 7 | 8
      mask TypeOptions slcdFormat: Decimal | Hex
      mask Display:
      | [data, map]=imread('LCD.gif');pic=ind2rgb(data,map);image(pic,[0.32 0.25 0.35 0.55]);
      | lineText = sprintf('Line %d', slcdLine);
      | text(0.5, 0.15, lineText, 'horizontalAlignment', 'center');
      | port_label('input', 1, '');
      | color('blue');
      | text(0.65, 0.87, 'LEGO', 'horizontalAlignment', 'left');
  P : Subsystem
  Reference : Subsystem
  Robot Tilt angle Set Point : Constant  Value=1.6  OutDataTypeStr=single
  Saturation2 : Saturate  UpperLimit=1  LowerLimit=0.45
  Sum1 : Sum  Inputs=|+-
  Sum2 : Sum  Inputs=|+-
  Sum3 : Sum
  Sum4 : Sum
  Sum5 : Sum  Inputs=+-
  Sum6 : Sum  Inputs=+-
  Switch : Switch
  tail : Outport  OutDataTypeStr=single  InitialOutput=0
  PWM_left : Outport  Port=2  OutDataTypeStr=single  InitialOutput=0
  PWM_right : Outport  Port=3  OutDataTypeStr=single  InitialOutput=0
  wires:
  Bus Selector/2 -> Gain2/1  "<battery>"
  Sum5/1 -> Switch/3  "tail"
  Dead Zone1/1 -> D/1(light error), P/1(light Error)
  Dead Zone/1 -> Gain1/1
  Demux/2 -> PWM_right/1, LCD1/1  "volt_right"
  Demux/1 -> PWM_left/1, LCD/1
  Switch/1 -> tail/1  "tail"
  sensors/1 -> Bus Selector/1
  Bus Selector/1 -> Sum1/2  "<light>"
  Saturation2/1 -> Sum2/2
  Sum1/1 -> Dead Zone1/1
  Sum4/1 -> Saturation2/1
  states/1 -> Bus Selector1/1
  Bus Selector1/1 -> Sum5/2  "<psi>"
  Robot Tilt angle Set Point/1 -> Sum5/1, Switch/1
  Constant1/1 -> Sum2/1
  lightCalib/1 -> Reference/1(calib)
  Reference/1(desired light) -> Sum1/1
  P/1(Volt) -> Sum4/1
  D/1(Volt) -> Sum4/2
  forwardSpeed/1 -> Sum6/1  "forward speed"
  Sum2/1 -> Gain/1
  Gain/1 -> Sum3/2
  Sum6/1 -> Sum3/1
  Gain1/1 -> Abs/1
  Bus Selector1/2 -> Dead Zone/1  "<phi_dot>"
  Abs/1 -> Sum6/2
  Sum3/1 -> Correction/1(VLVR)
  Correction/1(VLVRSAT) -> Demux/1
  Compare To Constant1/1 -> Switch/2
  Bus Selector1/3 -> Compare To Constant1/1  "<theta>"
  Gain2/1 -> LCD2/1(In1)

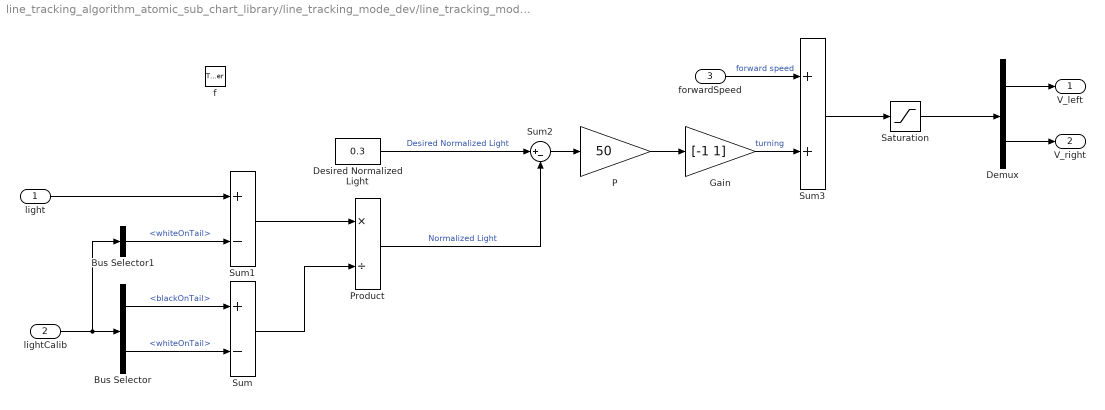
== system line_tracking_algorithm_atomic_sub_chart_library/line_tracking_mode_dev/line_tracking_mode.lineTrack ==
  light : Inport  OutDataTypeStr=single  PortDimensions=1
  lightCalib : Inport  Port=2  OutDataTypeStr=Bus: Light_Bus  PortDimensions=1
  forwardSpeed : Inport  Port=3  OutDataTypeStr=single  PortDimensions=1
  f : TriggerPort  TriggerType=function-call
      settings: CopyFcn=Stateflow.SLINSF.SimulinkMan.removeBlockPreDeleteFcn  PreDeleteFcn=Stateflow.SLINSF.SimulinkMan.unsafePredeleteFcn
  Bus Selector : BusSelector  OutputSignals=blackOnTail,whiteOnTail
  Bus Selector1 : BusSelector  OutputSignals=whiteOnTail
  Demux : Demux  Outputs=2
  Desired Normalized Light : Constant  Value=0.3  OutDataTypeStr=single
  Gain : Gain  Gain=[-1 1]
  P : Gain  Gain=50
  Product : Product  Inputs=*/
  Saturation : Saturate  UpperLimit=100  LowerLimit=-100  OutDataTypeStr=single
  Sum : Sum  Inputs=+-
  Sum1 : Sum  Inputs=+-
  Sum2 : Sum  Inputs=|+-
  Sum3 : Sum
  V_left : Outport  OutDataTypeStr=single  PortDimensions=1
  V_right : Outport  Port=2  OutDataTypeStr=single  PortDimensions=1
  wires:
  lightCalib/1 -> Bus Selector1/1, Bus Selector/1
  Bus Selector/2 -> Sum/2  "<whiteOnTail>"
  Bus Selector/1 -> Sum/1  "<blackOnTail>"
  Sum/1 -> Product/2
  light/1 -> Sum1/1
  Bus Selector1/1 -> Sum1/2  "<whiteOnTail>"
  Sum1/1 -> Product/1
  Product/1 -> Sum2/2  "Normalized Light"
  Desired Normalized Light/1 -> Sum2/1  "Desired Normalized Light"
  Sum2/1 -> P/1
  Gain/1 -> Sum3/2  "turning"
  Demux/1 -> V_left/1
  Demux/2 -> V_right/1
  forwardSpeed/1 -> Sum3/1  "forward speed"
  Sum3/1 -> Saturation/1
  P/1 -> Gain/1
  Saturation/1 -> Demux/1

== system line_tracking_algorithm_atomic_sub_chart_library/line_tracking_mode_dev/line_tracking_mode.tail_controller ==
  note: Could be improved, PI for example
  current : Inport  OutDataTypeStr=single  PortDimensions=1
  desired : Inport  Port=2  OutDataTypeStr=single  PortDimensions=1
  f : TriggerPort  TriggerType=function-call
      settings: CopyFcn=Stateflow.SLINSF.SimulinkMan.removeBlockPreDeleteFcn  PreDeleteFcn=Stateflow.SLINSF.SimulinkMan.unsafePredeleteFcn
  Gain : Gain  Gain=250
  Saturation : Saturate  UpperLimit=100  LowerLimit=-100  OutDataTypeStr=single
  Sum : Sum  Inputs=|+-
  cmd : Outport  OutDataTypeStr=single  PortDimensions=1  InitialOutput=0
  wires:
  Sum/1 -> Gain/1
  current/1 -> Sum/2
  desired/1 -> Sum/1
  Gain/1 -> Saturation/1
  Saturation/1 -> cmd/1

== system line_tracking_algorithm_atomic_sub_chart_library/line_tracking_mode_sid/line_tracking_mode.CalibrateLight ==
  light : Inport  OutDataTypeStr=single  PortDimensions=1
  lightCalib : Inport  Port=2  OutDataTypeStr=Bus: Light_Bus  PortDimensions=1
  f : TriggerPort  TriggerType=function-call
      settings: CopyFcn=Stateflow.SLINSF.SimulinkMan.removeBlockPreDeleteFcn  PreDeleteFcn=Stateflow.SLINSF.SimulinkMan.unsafePredeleteFcn
  Bus Selector : BusSelector  OutputSignals=blackOnTail,whiteOnTail
  Bus Selector1 : BusSelector  OutputSignals=whiteOnTail
  Product : Product  Inputs=*/
  Sum : Sum  Inputs=+-
  Sum1 : Sum  Inputs=+-
  CalibratedLight : Outport  OutDataTypeStr=single
  wires:
  Product/1 -> CalibratedLight/1  "Normalized Light"
  lightCalib/1 -> Bus Selector1/1, Bus Selector/1
  Bus Selector/2 -> Sum/2  "<whiteOnTail>"
  Bus Selector/1 -> Sum/1  "<blackOnTail>"
  Sum/1 -> Product/2
  light/1 -> Sum1/1
  Bus Selector1/1 -> Sum1/2  "<whiteOnTail>"
  Sum1/1 -> Product/1

== system line_tracking_algorithm_atomic_sub_chart_library/line_tracking_mode_sid/line_tracking_mode.Speak ==
  f : TriggerPort  TriggerType=function-call
      settings: CopyFcn=Stateflow.SLINSF.SimulinkMan.removeBlockPreDeleteFcn  PreDeleteFcn=Stateflow.SLINSF.SimulinkMan.unsafePredeleteFcn
  Constant : Constant  Value=50
  Speaker : legonxtlib/Speaker  sinputMode=Volume only  sspeakerFreq=800  sspeakerVolume=50  sspeakerDuration=100
  wires:
  Constant/1 -> Speaker/1

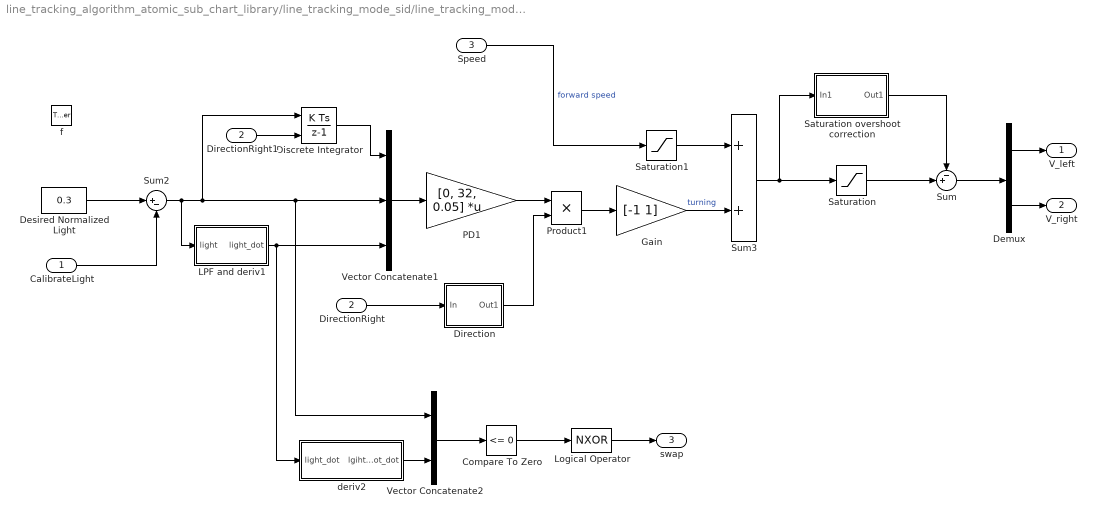
== system line_tracking_algorithm_atomic_sub_chart_library/line_tracking_mode_sid/line_tracking_mode.lineTrack ==
  CalibrateLight : Inport  OutDataTypeStr=single  PortDimensions=1
  DirectionRight : Inport  Port=2  OutDataTypeStr=boolean  PortDimensions=1
  Speed : Inport  Port=3  OutDataTypeStr=single  PortDimensions=1
  f : TriggerPort  TriggerType=function-call
      settings: CopyFcn=Stateflow.SLINSF.SimulinkMan.removeBlockPreDeleteFcn  PreDeleteFcn=Stateflow.SLINSF.SimulinkMan.unsafePredeleteFcn
  Compare To Zero : simulink/Logic and Bit Operations/Compare To Zero  relop=<=  OutDataTypeStr=boolean
  Demux : Demux  Outputs=2
  Desired Normalized Light : Constant  Value=0.3  OutDataTypeStr=single
  Direction : Subsystem
  DirectionRight1 : InportShadow  Port=2  OutDataTypeStr=boolean  PortDimensions=1
  Discrete Integrator : DiscreteIntegrator  gainval=0.1  ExternalReset=either  SampleTime=-1  IgnoreLimit=on  ICPrevOutput=DiscIntNeverNeededParam  ICPrevScaledInput=DiscIntNeverNeededParam
  Gain : Gain  Gain=[-1 1]
  LPF and deriv1 : Subsystem
  Logical Operator : Logic  Operator=NXOR  Inputs=1  AllPortsSameDT=off  OutDataTypeStr=boolean
  PD1 : Gain  Gain=[0, 32, 0.05]  Multiplication=Matrix(K*u)
  Product1 : Product
  Saturation : Saturate  UpperLimit=100  LowerLimit=-100  OutDataTypeStr=single
  Saturation overshoot correction : Subsystem
  Saturation1 : Saturate  UpperLimit=100  LowerLimit=40  OutDataTypeStr=single
  Sum : Sum  Inputs=-+|
  Sum2 : Sum  Inputs=|+-
  Sum3 : Sum
  Vector Concatenate1 : Concatenate  NumInputs=3
  Vector Concatenate2 : Concatenate
  deriv2 : Subsystem
  V_left : Outport  OutDataTypeStr=single  PortDimensions=1
  V_right : Outport  Port=2  OutDataTypeStr=single  PortDimensions=1
  swap : Outport  Port=3  OutDataTypeStr=boolean  PortDimensions=1
  wires:
  DirectionRight1/1 -> Discrete Integrator/2
  Saturation1/1 -> Sum3/1
  Speed/1 -> Saturation1/1  "forward speed"
  Discrete Integrator/1 -> Vector Concatenate1/1
  Sum2/1 -> Discrete Integrator/1, Vector Concatenate1/2, Vector Concatenate2/1, LPF and deriv1/1(light)
  Saturation overshoot correction/1(Out1) -> Sum/1
  Sum/1 -> Demux/1
  Saturation/1 -> Sum/2
  Vector Concatenate2/1 -> Compare To Zero/1
  Compare To Zero/1 -> Logical Operator/1
  deriv2/1(lgiht_dot_dot) -> Vector Concatenate2/2
  Logical Operator/1 -> swap/1
  LPF and deriv1/1(light_dot) -> Vector Concatenate1/3, deriv2/1(light_dot)
  Vector Concatenate1/1 -> PD1/1
  CalibrateLight/1 -> Sum2/2
  Desired Normalized Light/1 -> Sum2/1
  Direction/1(Out1) -> Product1/2
  DirectionRight/1 -> Direction/1(In)
  Product1/1 -> Gain/1
  Gain/1 -> Sum3/2  "turning"
  Demux/1 -> V_left/1
  Demux/2 -> V_right/1
  Sum3/1 -> Saturation overshoot correction/1(In1), Saturation/1
  PD1/1 -> Product1/1

== system line_tracking_algorithm_atomic_sub_chart_library/line_tracking_mode_sid/line_tracking_mode.phiController ==
  phi : Inport  OutDataTypeStr=single  PortDimensions=1
  desiredPhi : Inport  Port=2  OutDataTypeStr=single  PortDimensions=1
  battery : Inport  Port=3  OutDataTypeStr=double  PortDimensions=1
  f : TriggerPort  TriggerType=function-call
      settings: CopyFcn=Stateflow.SLINSF.SimulinkMan.removeBlockPreDeleteFcn  PreDeleteFcn=Stateflow.SLINSF.SimulinkMan.unsafePredeleteFcn
  Divide : Product  Inputs=*/
  Gain : Gain  Gain=-10
  Gain1 : Gain  Gain=100
  Saturation1 : Saturate  UpperLimit=100  LowerLimit=-100  OutDataTypeStr=single
  Sum : Sum  Inputs=|+-
  cmd : Outport  OutDataTypeStr=single
  wires:
  desiredPhi/1 -> Sum/1
  phi/1 -> Sum/2
  Sum/1 -> Gain/1
  battery/1 -> Divide/2
  Gain1/1 -> Saturation1/1
  Divide/1 -> Gain1/1
  Gain/1 -> Divide/1
  Saturation1/1 -> cmd/1

== system line_tracking_algorithm_atomic_sub_chart_library/line_tracking_mode_sid/line_tracking_mode.tail_controller ==
  note: Could be improved, PI for example
  current : Inport  OutDataTypeStr=single  PortDimensions=1
  desired : Inport  Port=2  OutDataTypeStr=single  PortDimensions=1
  f : TriggerPort  TriggerType=function-call
      settings: CopyFcn=Stateflow.SLINSF.SimulinkMan.removeBlockPreDeleteFcn  PreDeleteFcn=Stateflow.SLINSF.SimulinkMan.unsafePredeleteFcn
  Gain : Gain  Gain=250
  Saturation : Saturate  UpperLimit=100  LowerLimit=-100  OutDataTypeStr=single
  Sum : Sum  Inputs=|+-
  cmd : Outport  OutDataTypeStr=single  PortDimensions=1  InitialOutput=0
  wires:
  Sum/1 -> Gain/1
  current/1 -> Sum/2
  desired/1 -> Sum/1
  Gain/1 -> Saturation/1
  Saturation/1 -> cmd/1

== system line_tracking_algorithm_atomic_sub_chart_library/line_tracking_limbo/line_tracking_mode.LineTrackAltFcn/Correction ==
  VLVR : Inport
  Abs1 : Abs
  Compare To Constant1 : simulink/Logic and Bit Operations/Compare To Constant  relop=>  const=100  OutDataTypeStr=boolean
  Correction For Saturation : Subsystem  TreatAsAtomicUnit=on
  Logical Operator : Logic  Operator=OR  Inputs=1  AllPortsSameDT=off  OutDataTypeStr=boolean
  Logical Operator1 : Logic  Operator=NOT  Inputs=1  AllPortsSameDT=off  OutDataTypeStr=boolean
  Merge : Merge
  Multiply : Product  Inputs=**
  No saturation : Subsystem  TreatAsAtomicUnit=on
  Sign : Signum
  VLVRSAT : Outport
  wires:
  Multiply/1 -> VLVRSAT/1
  Sign/1 -> Multiply/1
  Merge/1 -> Multiply/2
  No saturation/1(Out1) -> Merge/2
  Correction For Saturation/1(Out1) -> Merge/1
  Logical Operator1/1 -> No saturation/Enable
  Logical Operator/1 -> Correction For Saturation/Enable, Logical Operator1/1
  Compare To Constant1/1 -> Logical Operator/1
  Abs1/1 -> Compare To Constant1/1, Correction For Saturation/1(In1), No saturation/1(In1)
  VLVR/1 -> Abs1/1, Sign/1

== system line_tracking_algorithm_atomic_sub_chart_library/line_tracking_limbo/line_tracking_mode.LineTrackAltFcn/D ==
  light error : Inport
  Abs1 : Abs
  Constant4 : Constant  Value=[3 0]  OutDataTypeStr=single
  Constant5 : Constant  Value=[0 1]  OutDataTypeStr=single
  Discrete Derivative1 : simulink/Discrete/Discrete Derivative  gainval=1.0  ICPrevScaledInput=0.0  InputProcessing=Inherited  OutMin=[]  OutMax=[]  OutDataTypeStr=single  OutputDataTypeScalingMode=single  OutDataType=fixdt(1, 16)  OutScaling=2^-10  DoSatur=off
  Gain2 : Gain  Gain=0.002
  Low Pass Filter1 : DiscreteFilter  Numerator=[.2]  Denominator=[1 -0.8]
  Product1 : Product  RndMeth=Zero
  Switch1 : Switch
  Volt : Outport
  wires:
  Product1/1 -> Volt/1
  Gain2/1 -> Product1/2
  Switch1/1 -> Product1/1
  Discrete Derivative1/1 -> Abs1/1, Switch1/2
  Constant4/1 -> Switch1/1
  Constant5/1 -> Switch1/3
  Abs1/1 -> Gain2/1
  Low Pass Filter1/1 -> Discrete Derivative1/1
  light error/1 -> Low Pass Filter1/1

== system line_tracking_algorithm_atomic_sub_chart_library/line_tracking_limbo/line_tracking_mode.LineTrackAltFcn/LCD2 ==
  In1 : Inport
  Data Type Conversion : DataTypeConversion  OutDataTypeStr=int32
  LCD : S-Function  FunctionName=nxt_lcd  Parameters=lcdStr1, lcdLine, lcdFormat  EnableBusSupport=off  mask(NXT LCD){lcdStr=Battery, lcdLine=8, lcdFormat=Decimal}
      mask prompts: lcdStr "Prefix String (MAX 8 Characters):"; lcdLine "Display at Line:"; lcdFormat "Display Format:"
      mask help: Displays a number on NXT LCD screen
      mask init:
      | lcdStr1= [uint8(lcdStr) uint8(0)];
      mask TypeOptions lcdLine: 1 | 2 | 3 | 4 | 5 | 6 | 7 | 8
      mask TypeOptions lcdFormat: Decimal | Hex
      mask Display:
      | color('blue');
      | text(0.65, 0.87, 'LEGO', 'horizontalAlignment', 'left');
      | color('black');
      | port_label('input', 1, '');
  wires:
  Data Type Conversion/1 -> LCD/1
  In1/1 -> Data Type Conversion/1

== system line_tracking_algorithm_atomic_sub_chart_library/line_tracking_limbo/line_tracking_mode.LineTrackAltFcn/P ==
  light Error : Inport
  Abs : Abs
  Constant2 : Constant  Value=[3 0]  OutDataTypeStr=single
  Constant3 : Constant  Value=[0 1]  OutDataTypeStr=single
  Gain4 : Gain  Gain=0.05
  Product : Product  RndMeth=Zero
  Switch : Switch
  Volt : Outport
  wires:
  Product/1 -> Volt/1
  Gain4/1 -> Product/2
  Abs/1 -> Gain4/1
  Constant2/1 -> Switch/1
  Constant3/1 -> Switch/3
  Switch/1 -> Product/1
  light Error/1 -> Switch/2, Abs/1

== system line_tracking_algorithm_atomic_sub_chart_library/line_tracking_limbo/line_tracking_mode.LineTrackAltFcn/Reference ==
  calib : Inport
  Bus Selector2 : BusSelector  OutputSignals=blackOnTail,whiteOnTail
  Gain : Gain  Gain=0.3
  Sum : Sum  Inputs=|+-
  Sum3 : Sum  Inputs=|++
  desired light : Outport
  wires:
  Sum3/1 -> desired light/1
  Gain/1 -> Sum3/1
  Sum/1 -> Gain/1
  Bus Selector2/1 -> Sum/1  "<blackOnTail>"
  Bus Selector2/2 -> Sum/2, Sum3/2  "<whiteOnTail>"
  calib/1 -> Bus Selector2/1

== system line_tracking_algorithm_atomic_sub_chart_library/line_tracking_mode/line_tracking_mode.LineTrackAltFcn/Correction ==
  VLVR : Inport
  Abs1 : Abs
  Compare To Constant1 : simulink/Logic and Bit Operations/Compare To Constant  relop=>  const=100  OutDataTypeStr=boolean
  Correction For Saturation : Subsystem  TreatAsAtomicUnit=on
  Logical Operator : Logic  Operator=OR  Inputs=1  AllPortsSameDT=off  OutDataTypeStr=boolean
  Logical Operator1 : Logic  Operator=NOT  Inputs=1  AllPortsSameDT=off  OutDataTypeStr=boolean
  Merge : Merge
  Multiply : Product  Inputs=**
  No saturation : Subsystem  TreatAsAtomicUnit=on
  Sign : Signum
  VLVRSAT : Outport
  wires:
  Multiply/1 -> VLVRSAT/1
  Sign/1 -> Multiply/1
  Merge/1 -> Multiply/2
  No saturation/1(Out1) -> Merge/2
  Correction For Saturation/1(Out1) -> Merge/1
  Logical Operator1/1 -> No saturation/Enable
  Logical Operator/1 -> Correction For Saturation/Enable, Logical Operator1/1
  Compare To Constant1/1 -> Logical Operator/1
  Abs1/1 -> Compare To Constant1/1, Correction For Saturation/1(In1), No saturation/1(In1)
  VLVR/1 -> Abs1/1, Sign/1

== system line_tracking_algorithm_atomic_sub_chart_library/line_tracking_mode/line_tracking_mode.LineTrackAltFcn/D ==
  light error : Inport
  Abs1 : Abs
  Constant4 : Constant  Value=[3 0]  OutDataTypeStr=single
  Constant5 : Constant  Value=[0 1]  OutDataTypeStr=single
  Discrete Derivative1 : simulink/Discrete/Discrete Derivative  gainval=1.0  ICPrevScaledInput=0.0  InputProcessing=Inherited  OutMin=[]  OutMax=[]  OutDataTypeStr=single  OutputDataTypeScalingMode=single  OutDataType=fixdt(1, 16)  OutScaling=2^-10  DoSatur=off
  Gain2 : Gain  Gain=0.002
  Low Pass Filter1 : DiscreteFilter  Numerator=[.2]  Denominator=[1 -0.8]
  Product1 : Product  RndMeth=Zero
  Switch1 : Switch
  Volt : Outport
  wires:
  Product1/1 -> Volt/1
  Gain2/1 -> Product1/2
  Switch1/1 -> Product1/1
  Discrete Derivative1/1 -> Abs1/1, Switch1/2
  Constant4/1 -> Switch1/1
  Constant5/1 -> Switch1/3
  Abs1/1 -> Gain2/1
  Low Pass Filter1/1 -> Discrete Derivative1/1
  light error/1 -> Low Pass Filter1/1

== system line_tracking_algorithm_atomic_sub_chart_library/line_tracking_mode/line_tracking_mode.LineTrackAltFcn/LCD2 ==
  In1 : Inport
  Data Type Conversion : DataTypeConversion  OutDataTypeStr=int32
  LCD : S-Function  FunctionName=nxt_lcd  Parameters=lcdStr1, lcdLine, lcdFormat  EnableBusSupport=off  mask(NXT LCD){lcdStr=Battery, lcdLine=8, lcdFormat=Decimal}
      mask prompts: lcdStr "Prefix String (MAX 8 Characters):"; lcdLine "Display at Line:"; lcdFormat "Display Format:"
      mask help: Displays a number on NXT LCD screen
      mask init:
      | lcdStr1= [uint8(lcdStr) uint8(0)];
      mask TypeOptions lcdLine: 1 | 2 | 3 | 4 | 5 | 6 | 7 | 8
      mask TypeOptions lcdFormat: Decimal | Hex
      mask Display:
      | color('blue');
      | text(0.65, 0.87, 'LEGO', 'horizontalAlignment', 'left');
      | color('black');
      | port_label('input', 1, '');
  wires:
  Data Type Conversion/1 -> LCD/1
  In1/1 -> Data Type Conversion/1

== system line_tracking_algorithm_atomic_sub_chart_library/line_tracking_mode/line_tracking_mode.LineTrackAltFcn/P ==
  light Error : Inport
  Abs : Abs
  Constant2 : Constant  Value=[3 0]  OutDataTypeStr=single
  Constant3 : Constant  Value=[0 1]  OutDataTypeStr=single
  Gain4 : Gain  Gain=0.05
  Product : Product  RndMeth=Zero
  Switch : Switch
  Volt : Outport
  wires:
  Product/1 -> Volt/1
  Gain4/1 -> Product/2
  Abs/1 -> Gain4/1
  Constant2/1 -> Switch/1
  Constant3/1 -> Switch/3
  Switch/1 -> Product/1
  light Error/1 -> Switch/2, Abs/1

== system line_tracking_algorithm_atomic_sub_chart_library/line_tracking_mode/line_tracking_mode.LineTrackAltFcn/Reference ==
  calib : Inport
  Bus Selector2 : BusSelector  OutputSignals=blackOnTail,whiteOnTail
  Gain : Gain  Gain=0.3
  Sum : Sum  Inputs=|+-
  Sum3 : Sum  Inputs=|++
  desired light : Outport
  wires:
  Sum3/1 -> desired light/1
  Gain/1 -> Sum3/1
  Sum/1 -> Gain/1
  Bus Selector2/1 -> Sum/1  "<blackOnTail>"
  Bus Selector2/2 -> Sum/2, Sum3/2  "<whiteOnTail>"
  calib/1 -> Bus Selector2/1
